simulink model "lab1_2"  (R2020a)
settings: Solver=VariableStepAuto  StartTime=0.0  StopTime=10.0  RelTol=10e-10  AbsTol=10e-10
values from neighbouring files (symbols this model uses):
  den1 = cell2mat(den1)    [lab1.m]
  num1 = cell2mat(num1)    [lab1.m]
undefined symbols (not defined in the file or in its folder): k
settings Model: Creator=paulosga  LastModifiedBy=paulosga
settings SolverCC: AutoScaleAbsTol=off

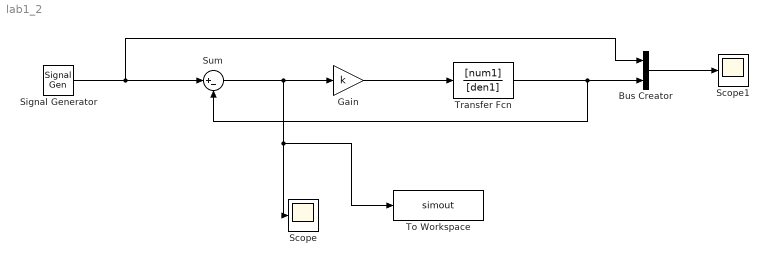
== system lab1_2 ==
  Bus Creator : BusCreator  Inputs=2
  Gain : Gain  Gain=k
  Scope : Scope
  Scope1 : Scope
  Signal Generator : SignalGenerator  WaveForm=square  Frequency=0.02
  Sum : Sum  Inputs=|+-
  To Workspace : ToWorkspace  VariableName=simout  SaveFormat=Timeseries  SampleTime=-1
  Transfer Fcn : TransferFcn  Numerator=[num1]  Denominator=[den1]
  wires:
  Signal Generator/1 -> Bus Creator/1, Sum/1
  Sum/1 -> To Workspace/1, Scope/1, Gain/1
  Gain/1 -> Transfer Fcn/1
  Transfer Fcn/1 -> Bus Creator/2, Sum/2
  Bus Creator/1 -> Scope1/1
